simulink model "controlSystem"  (R2021b)
settings: Solver=FixedStepDiscrete  StartTime=0.0  StopTime=10.0  FixedStep=5e-5  RelTol=1e-3
undefined symbols (not defined in the file): DiscIntNeverNeededParam, Reference, t_des
libraries: mcbcontrolslib x1
settings Model: Creator=andre  LastModifiedBy=andre

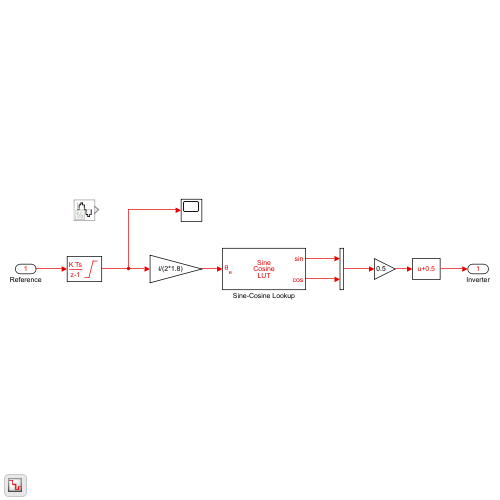
[thumbnail: Simulink's stored preview of the top-level diagram]
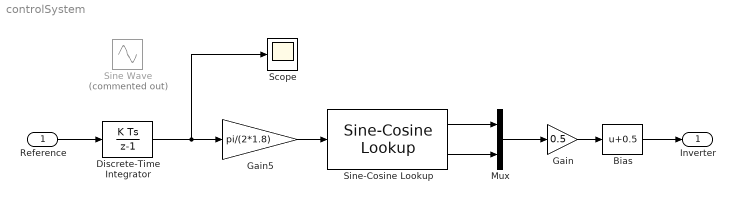
== system controlSystem ==
  Reference : Inport
  Bias : Bias  Bias=0.5
  Discrete-Time Integrator : DiscreteIntegrator  gainval=1/t_des  SampleTime=5e-5  LimitOutput=on  UpperSaturationLimit=Reference  LowerSaturationLimit=0  ICPrevOutput=DiscIntNeverNeededParam  ICPrevScaledInput=DiscIntNeverNeededParam
  Gain : Gain  Gain=0.5
  Gain5 : Gain  Gain=pi/(2*1.8)
  Mux : Mux  Inputs=2
  Scope : Scope
  Sine Wave : Sin  Commented=on  Amplitude=9  Frequency=2*pi*1  SampleTime=5e-5
  Sine-Cosine Lookup : mcbcontrolslib/Sine-Cosine Lookup  AngleInput=Radians  N_points=2048
      settings: SourceProductBaseCode=MT
  Inverter : Outport
  wires:
  Gain/1 -> Bias/1
  Gain5/1 -> Sine-Cosine Lookup/1
  Reference/1 -> Discrete-Time Integrator/1
  Bias/1 -> Inverter/1
  Discrete-Time Integrator/1 -> Gain5/1, Scope/1
  Mux/1 -> Gain/1
  Sine-Cosine Lookup/1 -> Mux/1
  Sine-Cosine Lookup/2 -> Mux/2
